simulink model "data_genrator_for_software_in_loop"  (R2025b)
settings: Solver=FixedStepDiscrete  StartTime=0.0  StopTime=150  FixedStep=2  RelTol=1e-3
libraries: dspstat3 x2
settings Model: Creator=Dell  LastModifiedBy=Dell

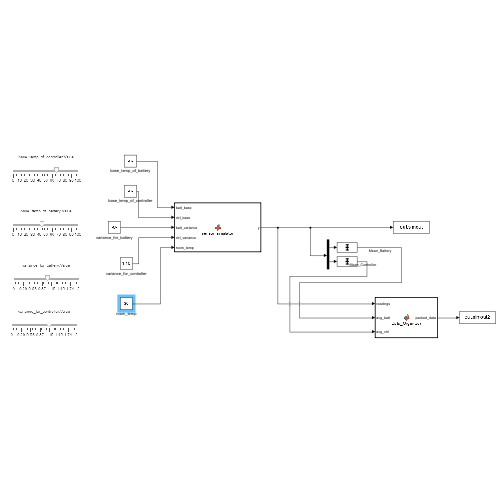
[thumbnail: Simulink's stored preview of the top-level diagram]
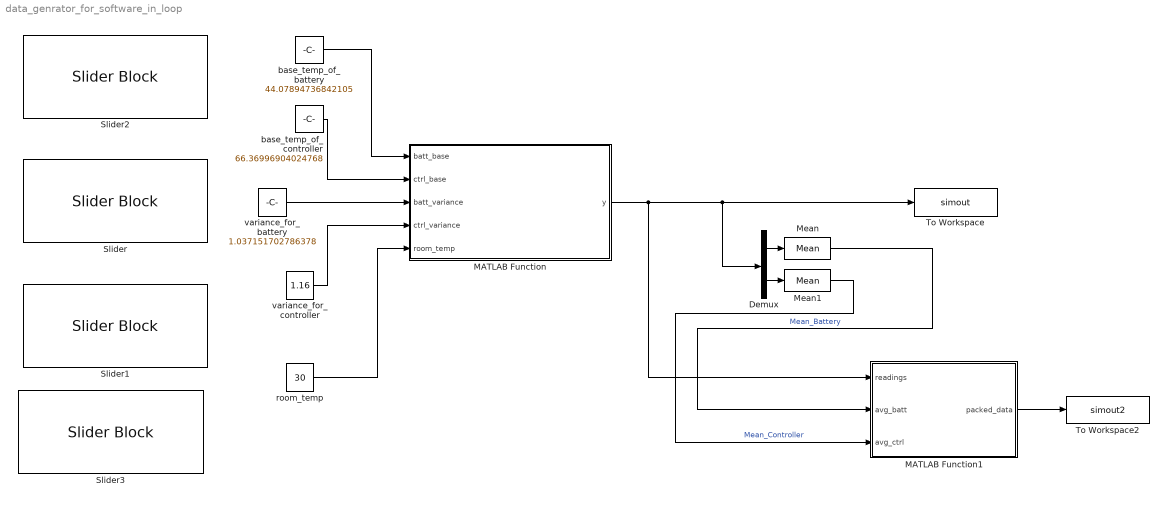
== system data_genrator_for_software_in_loop ==
  Demux : Demux  Outputs=[8,8]
  MATLAB Function : MATLAB Function  TreatAsAtomicUnit=on
  MATLAB Function1 : MATLAB Function  TreatAsAtomicUnit=on
  Mean : dspstat3/Mean  run=off  InputProcessing=Columns as channels (frame based)  reset_popup=None  directionMode=Each column  dimension=1  roiEnable=off  roiType=Rectangles  roiPortion=Entire ROI  roiOutput=Individual statistics for each ROI  roiFlag=off  roundingMode=Floor  overflowMode=off  outputDataTypeStr=Inherit: Same as accumulator  outputMin=[]  outputMax=[]  outputLastDataTypeStr=Inherit: Same as accumulator
  Mean1 : dspstat3/Mean  run=off  InputProcessing=Columns as channels (frame based)  reset_popup=None  directionMode=Each column  dimension=1  roiEnable=off  roiType=Rectangles  roiPortion=Entire ROI  roiOutput=Individual statistics for each ROI  roiFlag=off  roundingMode=Floor  overflowMode=off  outputDataTypeStr=Inherit: Same as accumulator  outputMin=[]  outputMax=[]  outputLastDataTypeStr=Inherit: Same as accumulator
  Slider : SliderBlock
  Slider1 : SliderBlock  ScaleMax=2
  Slider2 : SliderBlock
  Slider3 : SliderBlock  ScaleMax=2
  To Workspace : ToWorkspace  VariableName=simout  SaveFormat=Timeseries  SampleTime=-1
  To Workspace2 : ToWorkspace  VariableName=simout2  SampleTime=-1
  base_temp_of_battery : Constant  Value=44.07894736842105
  base_temp_of_controller : Constant  Value=66.36996904024768
  room_temp : Constant  Value=30
  variance_for_battery : Constant  Value=1.037151702786378
  variance_for_controller : Constant  Value=1.16
  wires:
  MATLAB Function/1(y) -> MATLAB Function1/1(readings), Demux/1, To Workspace/1
  base_temp_of_battery/1 -> MATLAB Function/1(batt_base)
  variance_for_battery/1 -> MATLAB Function/3(batt_variance)
  MATLAB Function1/1(packed_data) -> To Workspace2/1
  Demux/1 -> Mean/1
  Demux/2 -> Mean1/1
  Mean/1 -> MATLAB Function1/2(avg_batt)  "Mean_Battery"
  Mean1/1 -> MATLAB Function1/3(avg_ctrl)  "Mean_Controller"
  base_temp_of_controller/1 -> MATLAB Function/2(ctrl_base)
  variance_for_controller/1 -> MATLAB Function/4(ctrl_variance)
  room_temp/1 -> MATLAB Function/5(room_temp)

== matlab function data_genrator_for_software_in_loop/MATLAB Function1 ==
  data: readings input; packed_data output; avg_batt input; avg_ctrl input
function packed_data = Data_Organizer(readings, avg_batt, avg_ctrl)
    % readings: 16x1 vector from the sensor_simulator block
    % avg_batt: 1x1 scalar average from Mean_Battery
    % avg_ctrl: 1x1 scalar average from Mean_Controller
    
    % Core hardware tracking addresses
    addresses = [101:108, 201:208]'; 
    
    % Create a customized 16x1 average column:
    % The first 8 rows get assigned the Battery Average
    % The next 8 rows get assigned the Controller Average
    component_averages = [repmat(avg_batt, 8, 1); repmat(avg_ctrl, 8, 1)];
    
    % Combine into a single matrix [Address, Input Reading, Component-Specific Average]
    packed_data = [addresses, readings, component_averages];
end

== matlab function data_genrator_for_software_in_loop/MATLAB Function ==
  data: batt_base input; y output; ctrl_base input; batt_variance input; ctrl_variance input; room_temp input
function y = sensor_simulator(batt_base, ctrl_base, batt_variance, ctrl_variance, room_temp)
    % batt_base: Target temp for battery (Slider 1)
    % ctrl_base: Target temp for controller (Slider 2)
    % batt_variance: Noise % for battery (Slider 3, e.g., 2 for 2%)
    % ctrl_variance: Noise % for controller (Slider 4, e.g., 6 for 6%)
    % room_temp: Starting ambient temperature from external constant block
    
    % Track internal thermal buildup over time
    persistent thermal_step;
    if isempty(thermal_step)
        thermal_step = 0;
    end
    
    % Increment time steps dynamically to simulate thermodynamic inertia
    thermal_step = thermal_step + 0.05; 
    warmup_factor = 1 - exp(-thermal_step);
    
    % Calculate the dynamic, rising core profiles based on dynamic room_temp
    current_batt_center = room_temp + (batt_base - room_temp) * warmup_factor;
    current_ctrl_center = room_temp + (ctrl_base - room_temp) * warmup_factor;
    
    % Convert the 0-10 slider inputs to decimal percentages
    dec_batt_var = batt_variance / 100;
    dec_ctrl_var = ctrl_variance / 100;
    
    % Generate 16 completely independent random factors between -1 and 1
    random_factors = (2 * rand(16, 1) - 1);
    
    % Initialize our 16x1 tracking array
    y = zeros(16, 1);
    
    % --- 1. BATTERY SUB-ARRAY (Sensors 1 to 8) ---
    max_batt_offset = current_batt_center * dec_batt_var;
    y(1:8) = current_batt_center + (random_factors(1:8) * max_batt_offset);
    
    % --- 2. CONTROLLER SUB-ARRAY (Sensors 9 to 16) ---
    max_ctrl_offset = current_ctrl_center * dec_ctrl_var;
    y(9:16) = current_ctrl_center + (random_factors(9:16) * max_ctrl_offset);
end
